simulink model "StabilisationBF"  (R2017a)
settings: Solver=ode4  StartTime=0.0  StopTime=500  FixedStep=0.0001  RelTol=1e-3
values from neighbouring files (symbols this model uses):
  K = NaN    [FctPP.m]    (also in Gainfind.m; GainfindV2.m; GainfindVTD.m = struct('matrix',{zeros(m,n)}); Mainscript.m = cat(3,K(1:r).matrix))
  Parametres = [ax, bx, Rap, alpha, tau]    [Model.m]
  Parametres2 = [tr, f]    [Model.m]
settings Model: Creator=MONCEF  LastModifiedBy=MONCEF

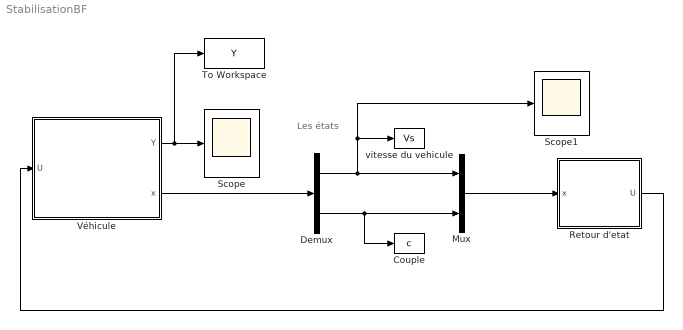
== system StabilisationBF ==
  note: Les états
  Couple : ToWorkspace  VariableName=c  SaveFormat=Structure With Time  SampleTime=0.001
  Demux : Demux  Outputs=2
  Mux : Mux  Inputs=2
  Retour d'etat : Subsystem
      mask Display: image(fullfile(pwd,'Images','Retour d''état (-).png'));
  Scope : Scope
  Scope1 : Scope
  To Workspace : ToWorkspace  VariableName=Y  SaveFormat=Structure With Time  SampleTime=0.001
  Véhicule : Subsystem
      mask Display: image(fullfile(pwd,'Images','VehiculeSuiveur.jpg'));
  vitesse du vehicule : ToWorkspace  VariableName=Vs  SaveFormat=Structure With Time  SampleTime=0.001
  wires:
  Véhicule/1(Y) -> To Workspace/1, Scope/1
  Demux/1 -> Mux/1, vitesse du vehicule/1, Scope1/1
  Demux/2 -> Mux/2, Couple/1
  Véhicule/2(x) -> Demux/1
  Retour d'etat/1(U) -> Véhicule/1(U)
  Mux/1 -> Retour d'etat/1(x)

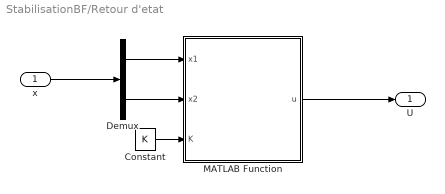
== system StabilisationBF/Retour d'etat ==
  x : Inport
  Constant : Constant  Value=K
  Demux : Demux  Outputs=2
  MATLAB Function : MATLAB Function  TreatAsAtomicUnit=on
  U : Outport
  wires:
  x/1 -> Demux/1
  MATLAB Function/1(u) -> U/1
  Constant/1 -> MATLAB Function/3(K)
  Demux/1 -> MATLAB Function/1(x1)
  Demux/2 -> MATLAB Function/2(x2)

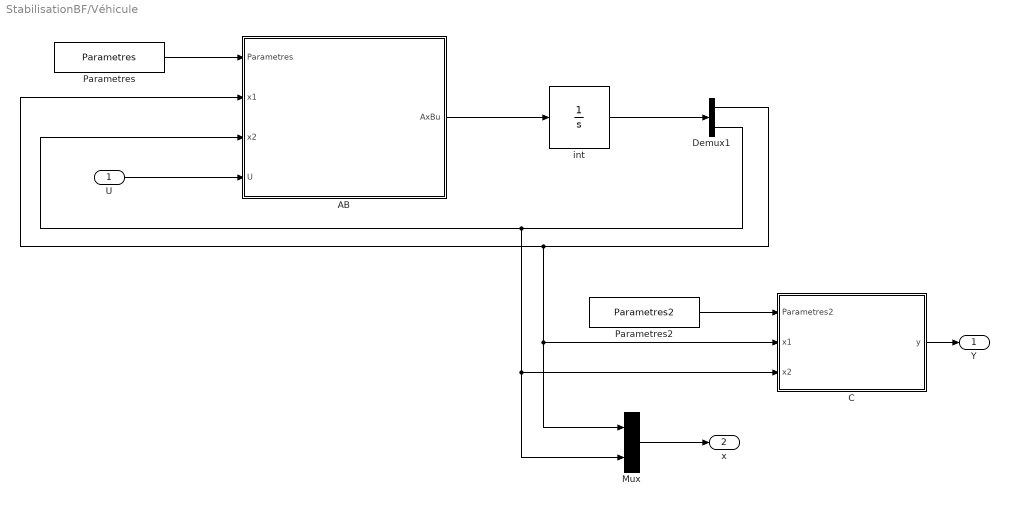
== system StabilisationBF/Véhicule ==
  U : Inport
  AB : MATLAB Function  TreatAsAtomicUnit=on
  C : MATLAB Function  TreatAsAtomicUnit=on
  Demux1 : Demux  Outputs=2
  Mux : Mux  Inputs=2
  Parametres : Constant  Value=Parametres
  Parametres2 : Constant  Value=Parametres2
  int : Integrator  InitialCondition=[10 0]
      mask Display: image(fullfile(pwd,'Images','Integrateur.png'));
  Y : Outport
  x : Outport  Port=2
  wires:
  C/1(y) -> Y/1
  Parametres/1 -> AB/1(Parametres)
  Parametres2/1 -> C/1(Parametres2)
  U/1 -> AB/4(U)
  AB/1(AxBu) -> int/1
  Demux1/2 -> Mux/2, C/3(x2), AB/3(x2)
  Demux1/1 -> Mux/1, C/2(x1), AB/2(x1)
  Mux/1 -> x/1
  int/1 -> Demux1/1

== matlab function StabilisationBF/Véhicule/AB ==
  data: Parametres input; x1 input; AxBu output; x2 input; U input
function AxBu = fcn(Parametres,x1,x2,U)

ax = Parametres(1);
bx = Parametres(2);
Rap = Parametres(3);
alpha = Parametres(4);
tau = Parametres(5);

%define the systeme matrix
A =[-(ax+bx*x1)/alpha Rap/alpha; 0 -1/tau];
B =[0 ; 1/tau];



AxBu = A*[x1;x2]+B*U;

== matlab function StabilisationBF/Retour d'etat/MATLAB Function ==
  data: x1 input; u output; x2 input; K input
function u = fcn(x1,x2,K)

x=[x1;x2];
K1=K(:,:,1);
K2=K(:,:,2);



T1 =(x1-0)/(100);
T2 =(100-x1)/(100);

u =-(T1*K1+T2*K2)*x;

== matlab function StabilisationBF/Véhicule/C ==
  data: Parametres2 input; x1 input; y output; x2 input
function y = fcn(Parametres2,x1,x2)
tr = Parametres2(1);
f = Parametres2(2);

C = [tr+f*x1 0];
y =C*[x1;x2];
